simulink model "sensor_model"  (R2026a)
settings: Solver=VariableStepAuto
undefined symbols (not defined in the file): engine

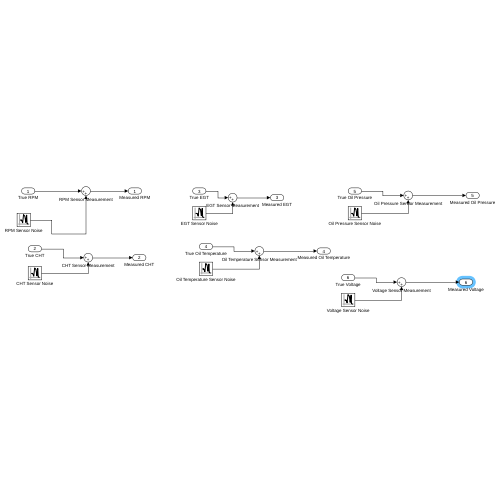
[thumbnail: Simulink's stored preview of the top-level diagram]
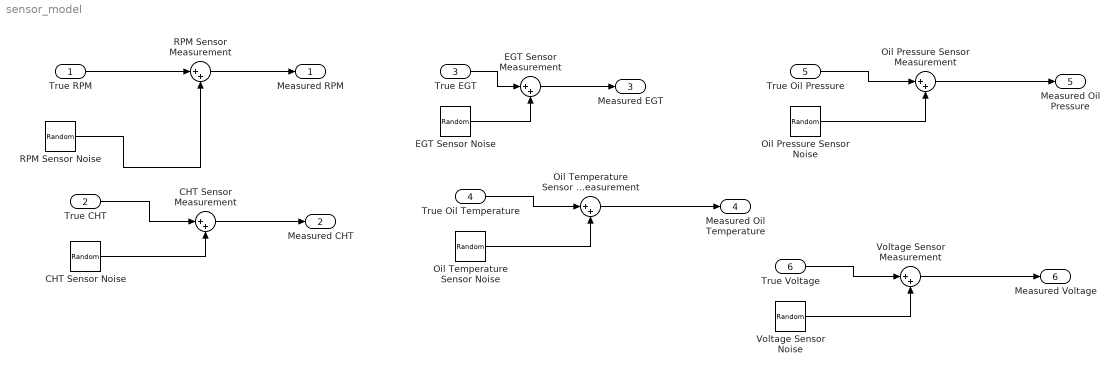
== system sensor_model ==
  True RPM : Inport
  True CHT : Inport  Port=2
  True EGT : Inport  Port=3
  True Oil Temperature : Inport  Port=4
  True Oil Pressure : Inport  Port=5
  True Voltage : Inport  Port=6
  CHT Sensor Measurement : Sum  Inputs=|++
  CHT Sensor Noise : RandomNumber  Mean=engine.chtSensorNoiseMean  Variance=engine.chtSensorNoiseVariance  Seed=23456  SampleTime=1
  EGT Sensor Measurement : Sum  Inputs=|++
  EGT Sensor Noise : RandomNumber  Mean=engine.egtSensorNoiseMean  Variance=engine.egtSensorNoiseVariance  Seed=34567  SampleTime=1
  Oil Pressure Sensor Measurement : Sum  Inputs=|++
  Oil Pressure Sensor Noise : RandomNumber  Mean=engine.oilPressureSensorNoiseMean  Variance=engine.oilPressureSensorNoiseVariance  Seed=56789  SampleTime=1
  Oil Temperature Sensor Measurement : Sum  Inputs=|++
  Oil Temperature Sensor Noise : RandomNumber  Mean=engine.oilTempSensorNoiseMean  Variance=engine.oilTempSensorNoiseVariance  Seed=45678  SampleTime=1
  RPM Sensor Measurement : Sum  Inputs=|++
  RPM Sensor Noise : RandomNumber  Mean=engine.rpmSensorNoiseMean  Variance=engine.rpmSensorNoiseVariance  Seed=12345  SampleTime=1
  Voltage Sensor Measurement : Sum  Inputs=|++
  Voltage Sensor Noise : RandomNumber  Mean=engine.voltageSensorNoiseMean  Variance=engine.voltageSensorNoiseVariance  Seed=67890  SampleTime=1
  Measured RPM : Outport
  Measured CHT : Outport  Port=2
  Measured EGT : Outport  Port=3
  Measured Oil Temperature : Outport  Port=4
  Measured Oil Pressure : Outport  Port=5
  Measured Voltage : Outport  Port=6
  wires:
  RPM Sensor Noise/1 -> RPM Sensor Measurement/2
  True RPM/1 -> RPM Sensor Measurement/1
  RPM Sensor Measurement/1 -> Measured RPM/1
  True CHT/1 -> CHT Sensor Measurement/1
  CHT Sensor Noise/1 -> CHT Sensor Measurement/2
  CHT Sensor Measurement/1 -> Measured CHT/1
  True EGT/1 -> EGT Sensor Measurement/1
  EGT Sensor Noise/1 -> EGT Sensor Measurement/2
  EGT Sensor Measurement/1 -> Measured EGT/1
  Oil Temperature Sensor Noise/1 -> Oil Temperature Sensor Measurement/2
  True Oil Temperature/1 -> Oil Temperature Sensor Measurement/1
  Oil Temperature Sensor Measurement/1 -> Measured Oil Temperature/1
  True Oil Pressure/1 -> Oil Pressure Sensor Measurement/1
  Oil Pressure Sensor Measurement/1 -> Measured Oil Pressure/1
  Oil Pressure Sensor Noise/1 -> Oil Pressure Sensor Measurement/2
  True Voltage/1 -> Voltage Sensor Measurement/1
  Voltage Sensor Measurement/1 -> Measured Voltage/1
  Voltage Sensor Noise/1 -> Voltage Sensor Measurement/2
